simulink model "audiolatencymeasurement"  (R2014a)
settings: Solver=FixedStepDiscrete  StartTime=0.0  StopTime=inf  FixedStep=1/44100  RelTol=1e-3
libraries: dspsrcs4 x1, dspvision x1, dspsnks4 x1
settings Model: Creator=The MathWorks Inc.
settings DebuggingCC: UnderspecifiedInitializationDetection=Classic

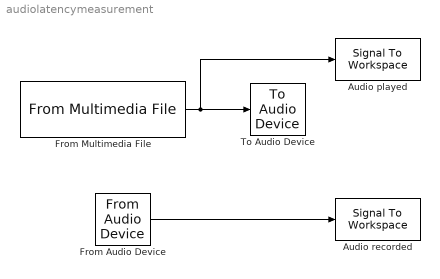
== system audiolatencymeasurement ==
  Audio played : SignalToWorkspace  VariableName=audioOut
      settings: CopyFcn=dspblkcopystw(gcbh);
  Audio recorded : SignalToWorkspace  VariableName=audioIn
      settings: CopyFcn=dspblkcopystw(gcbh);
  From Audio Device : dspsrcs4/From Audio Device  deviceName=Default  numChannels=2  sampleRate=44100  deviceDatatype=Determine from output data type  autoBufferSize=on  bufferSize=4096  queueDuration=1.0  frameSize=1024  outputDatatype=double  defaultInputChannelMapping=on  inputChannelMapping=1:2
  From Multimedia File : dspvision/From Multimedia File  inputFilename=guitar10min.ogg  loop=on  numPlays=inf  outputStreams=Audio only  videoDataType=single  audioDataType=double  inheritSampleTime=on  userDefinedSampleTime=1/30  noAudioOutput=off  isIntensityVideo=off  fourcc=RGB  colorVideoFormat=Separate color signals  outputEOF=off  dataOrg=Column-major  audioFrameSize=1024  computeAudioFrameSize=off  outSamplingMode=Frame based
  To Audio Device : dspsnks4/To Audio Device  deviceName=Default  inheritSampleRate=on  sampleRate=44100  deviceDatatype=Determine from input data type  autoBufferSize=on  bufferSize=4096  queueDuration=1.0  defaultOutputChannelMapping=on  outputChannelMapping=1:2
  wires:
  From Multimedia File/1 -> To Audio Device/1, Audio played/1
  From Audio Device/1 -> Audio recorded/1
